simulink model "w1p8"  (R2020b)
settings: Solver=VariableStepAuto  StartTime=0.0  StopTime=10.0  RelTol=1e-3
settings Model: Creator=Dell  LastModifiedBy=Dell

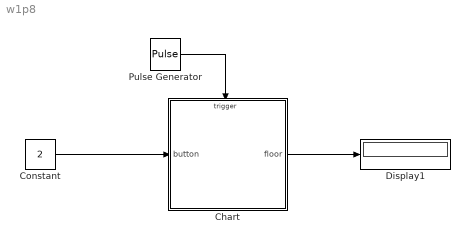
== system w1p8 ==
  Chart : Stateflow chart  TreatAsAtomicUnit=on
  Constant : Constant  Value=2
  Display1 : Display
  Pulse Generator : DiscretePulseGenerator  PulseType=Time based  Period=10  PulseWidth=5
  wires:
  Constant/1 -> Chart/1(button)
  Chart/1(floor) -> Display1/1
  Pulse Generator/1 -> Chart/Trigger

== stateflow chart w1p8/Chart ==
  settings: executeAtInitialization=1
  state Idle
  state Initial
    en:
    door_close=1;
  state Lift_work
    state Run [parallel]
      settings: executionOrder=1
      state Floor1
        en:
        floor=1;
        (default) -> (junction 17)
        (junction 17) -> (junction 18) [order 1] : [floor==button]
        (junction 17) -> (junction 19) [order 2]
        (junction 18) -> (junction 20) : {door_close=0;}/{delay.cnt}
        (junction 20) -> (junction 19)
        (junction 19) -> (junction 21)
      state Floor2
        en:
        floor=2;
        (default) -> (junction 30)
        (junction 30) -> (junction 31) [order 1] : [floor==button]
        (junction 30) -> (junction 32) [order 2]
        (junction 31) -> (junction 33) : {door_close=0;}/{delay.cnt}
        (junction 33) -> (junction 32)
        (junction 32) -> (junction 34)
      state Floor3
        en:
        floor=3;
        (default) -> (junction 42)
        (junction 42) -> (junction 43) [order 1] : [floor==button]
        (junction 42) -> (junction 44) [order 2]
        (junction 43) -> (junction 45) : {door_close=0;}/{delay.cnt}
        (junction 45) -> (junction 44)
        (junction 44) -> (junction 46)
      state Floor4
        en:
        floor=4;
        (default) -> (junction 54)
        (junction 54) -> (junction 55) [order 1] : [floor==button]
        (junction 54) -> (junction 56) [order 2]
        (junction 55) -> (junction 57) : {door_close=0;}/{delay.cnt}
        (junction 57) -> (junction 56)
        (junction 56) -> (junction 58)
      state Floor5
        en:
        floor=5;
        (default) -> (junction 66)
        (junction 66) -> (junction 67) [order 1] : [floor==button]
        (junction 66) -> (junction 68) [order 2]
        (junction 67) -> (junction 69) : {door_close=0;}/{delay.cnt}
        (junction 69) -> (junction 68)
        (junction 68) -> (junction 70)
      (default) -> Floor1
      Floor2 -> Floor1 [order 2] : [button<floor]
      Floor1 -> Floor2 : [button>floor]
      Floor3 -> Floor2 [order 2] : [button<floor]
      Floor2 -> Floor3 [order 1] : [button>floor]
      Floor4 -> Floor3 [order 2] : [button<floor]
      Floor3 -> Floor4 [order 1] : [button>floor]
      Floor5 -> Floor4 : [button<floor]
      Floor4 -> Floor5 [order 1] : [button>floor]
    state delay [parallel]
      settings: executionOrder=2
      state init
        en:
        d=0;
      state Hold
        du:
        d=d+1;
      (default) -> init
      Hold -> init : [d>5]{door_close=1}
      init -> Hold : cnt
  (default) -> Idle
  Lift_work -> Idle : [door_close==1 && floor == button]
  Idle -> Initial : request
  Initial -> Lift_work
  data: button input; floor output; door_close local; d local
  events: cnt local FUNCTION_CALL_EVENT; request input RISING_EDGE_EVENT
